simulink library "KepOrbit"  (R2014b)
settings: Solver=VariableStepAuto  StartTime=0.0  StopTime=10.0  RelTol=1e-3
undefined symbols (not defined in the file or in its folder): ConfParam
settings Model: Creator=p.cruciani  LastModifiedBy=Hp
settings DataIOCC: SaveFormat=Dataset
settings OptimizationCC: UseDivisionForNetSlopeComputation=off  SimCompilerOptimization=off
settings DebuggingCC: SolverPrmCheckMsg=none  FrameProcessingCompatibilityMsg=error  AllowSymbolicDim=off
settings HardwareCC: ProdBitPerPointer=64  ProdLargestAtomicFloat=Float  ProdIntDivRoundTo=Zero  ProdEndianess=LittleEndian  ProdWordSize=64  ProdHWDeviceType=Intel->x86-64 (Windows64)
settings RTWCC: RTWCompilerOptimization=off
settings GRTTargetCC: GeneratePreprocessorConditionals=Use local settings
settings ConfigComp: CovMetricSettings=dw  CovHtmlReporting=on  CovSaveCumulativeToWorkspaceVar=on  CovSaveSingleToWorkspaceVar=on  CovExternalEMLEnable=off

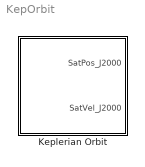
== system KepOrbit ==
  Keplerian Orbit : Subsystem

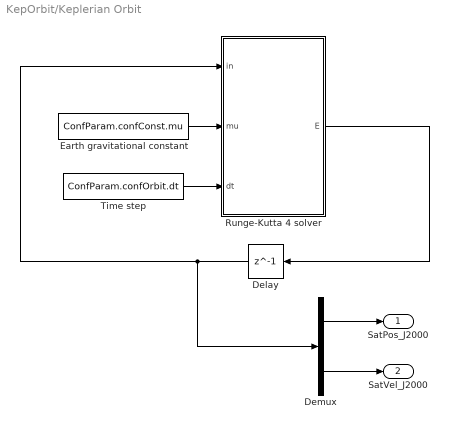
== system KepOrbit/Keplerian Orbit ==
  Delay : Delay  DelayLength=1  InitialCondition=ConfParam.confOrbit.InitOrbit  SampleTime=ConfParam.confOrbit.dt
  Demux : Demux  Outputs=2
  Earth gravitational constant : Constant  Value=ConfParam.confConst.mu
  Runge-Kutta 4 solver : MATLAB Function  TreatAsAtomicUnit=on
  Time step : Constant  Value=ConfParam.confOrbit.dt
  SatPos_J2000 : Outport
  SatVel_J2000 : Outport  Port=2
  wires:
  Runge-Kutta 4 solver/1(E) -> Delay/1
  Earth gravitational constant/1 -> Runge-Kutta 4 solver/2(mu)
  Time step/1 -> Runge-Kutta 4 solver/3(dt)
  Delay/1 -> Demux/1, Runge-Kutta 4 solver/1(in)
  Demux/1 -> SatPos_J2000/1
  Demux/2 -> SatVel_J2000/1

== matlab function KepOrbit/Keplerian Orbit/Runge-Kutta 4 solver ==
  data: in input; E output; mu input; dt input
function E=RK4(in,mu,dt)
    % Runge-Kutta 4 solver      
    E=in;
    Ei=in;
    
    K1=dyn_kin(Ei,mu);
    
    Ei(:)=E(:)+dt/2*K1;
    K2=dyn_kin(Ei,mu);
    
    Ei(:)=E(:)+dt/2*K2;
    K3=dyn_kin(Ei,mu);
    
    Ei(:)=E(:)+dt*K3;
    K4=dyn_kin(Ei,mu);
    
    E(:)=E(:)+dt/6*(K1+2*(K2+K3)+K4);

end
